simulink model "tsl235r_freq"  (R2013b)
settings: Solver=ode45  StartTime=0.0  StopTime=10.0  RelTol=1e-3
settings Model: Creator=Markus  LastModifiedBy=Markus

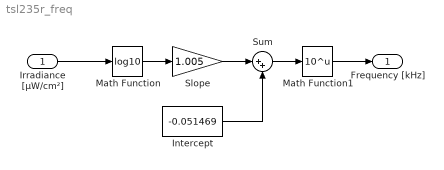
== system tsl235r_freq ==
  Irradiance [µW/cm²] : Inport
  Intercept : Constant  Value=-0.051469
  Math Function : Math  Operator=log10  SaturateOnIntegerOverflow=on
  Math Function1 : Math  Operator=10^u  SaturateOnIntegerOverflow=on
  Slope : Gain  Gain=1.005
  Sum : Sum  Inputs=|++
  Frequency [kHz] : Outport
  wires:
  Irradiance [µW/cm²]/1 -> Math Function/1
  Math Function/1 -> Slope/1
  Slope/1 -> Sum/1
  Intercept/1 -> Sum/2
  Sum/1 -> Math Function1/1
  Math Function1/1 -> Frequency [kHz]/1
